simulink model "sim_linear_stateObserver"  (R2020a)
settings: Solver=ode4  StartTime=0.0  StopTime=inf  FixedStep=0.01  RelTol=1e-3
InitFcn:
  | run('initialize_system.m')
values from neighbouring files (symbols this model uses):
  Ac = [d_f1_dth,d_f1_dyw,d_f1_dw_th,d_f1_dw_yw ... (first row only)    [linearize_heli.m]
  Bc = [d_f1_Vmp,d_f1_Vmy ... (first row only)    [linearize_heli.m]
  Cc = [1,0,0,0;0,1,0,0]    [linearize_heli.m]
  th_op = -30*pi/180    (= -0.523598775598)    [initialize_system.m]
  Vmp_op = (Kyy*m_heli*g*cos(th_op)*l_cm) / (Kyy*Kpp - Kyp*Kpy)    [initialize_system.m]
  Vmy_op = (Kyp*Vmp_op) / (Kyy)    [initialize_system.m]
  w_th_op = 0    [initialize_system.m]
  w_yw_op = 0    [initialize_system.m]
  yw_op = pi/2    (= 1.57079632679)    [initialize_system.m]
undefined symbols (not defined in the file or in its folder): L
libraries: realtime_pacer_lib x1
settings Model: Creator=engen  LastModifiedBy=eirik.engen

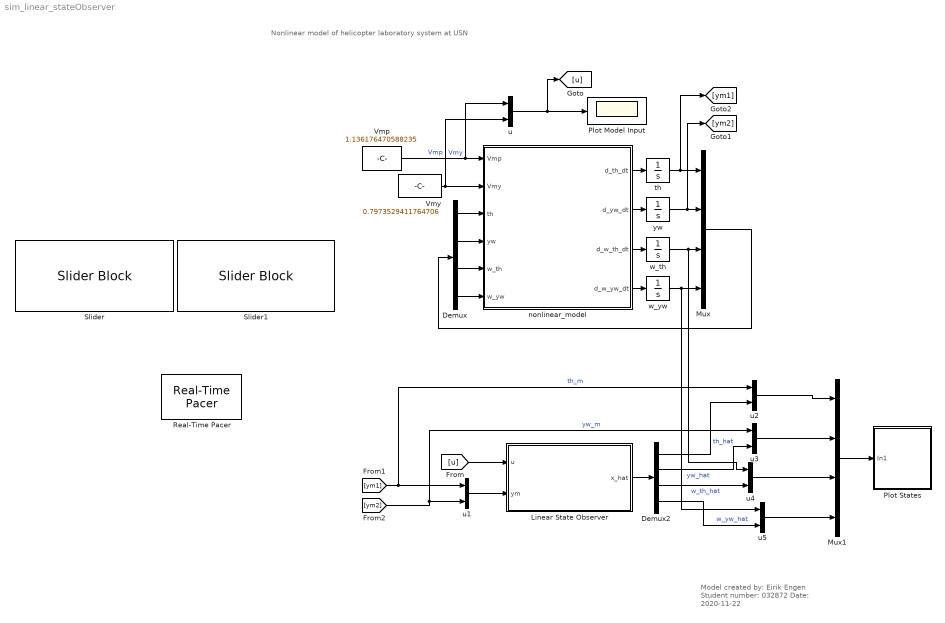
== system sim_linear_stateObserver ==
  note: Model created by: Eirik Engen
      | Student number: 032872
      | Date: 2020-11-22
  note: Nonlinear model of helicopter laboratory system at USN
  Demux : Demux
  Demux2 : Demux
  Linear State Observer : Subsystem
  Mux : Mux
  Mux1 : Mux
  Plot Model Input : Scope
  Plot States : Subsystem
  Real-Time Pacer : realtime_pacer_lib/Real-Time Pacer  simTimePerRealTime=1
      settings: SourceProductName=Real-Time Pacer
  Slider : SliderBlock  ScaleMax=1.6  TickInterval=0.4
  Slider1 : SliderBlock  ScaleMax=1.6  TickInterval=0.4
  Vmp : Constant  Value=1.136176470588235  SampleTime=-1
  Vmy : Constant  Value=0.7973529411764706  SampleTime=-1
  nonlinear_model : MATLAB Function  TreatAsAtomicUnit=on
  th : Integrator  InitialCondition=-10*pi/180  LimitOutput=on  UpperSaturationLimit=45*pi/180  LowerSaturationLimit=-45*pi/180  ContinuousStateAttributes='th'
  u{,1..5} (6 alike) : Mux  Inputs=2
  w_th : Integrator  ContinuousStateAttributes='w_th'
  w_yw : Integrator  ContinuousStateAttributes='w_yw'
  yw : Integrator  InitialCondition=pi/2  LimitOutput=on  UpperSaturationLimit=180*pi/180  LowerSaturationLimit=0  ContinuousStateAttributes='yw'
  wires:
  Vmp/1 -> u/1, nonlinear_model/1(Vmp)  "Vmp"
  Vmy/1 -> u/2, nonlinear_model/2(Vmy)  "Vmy"
  nonlinear_model/1(d_th_dt) -> th/1
  nonlinear_model/2(d_yw_dt) -> yw/1
  nonlinear_model/3(d_w_th_dt) -> w_th/1
  nonlinear_model/4(d_w_yw_dt) -> w_yw/1
  th/1 -> [ym1], Mux/1
  yw/1 -> [ym2], Mux/2
  w_th/1 -> u4/1, Mux/3
  w_yw/1 -> u5/1, Mux/4
  Mux/1 -> Demux/1
  Demux/1 -> nonlinear_model/3(th)
  Demux/2 -> nonlinear_model/4(yw)
  Demux/3 -> nonlinear_model/5(w_th)
  Demux/4 -> nonlinear_model/6(w_yw)
  u/1 -> [u], Plot Model Input/1
  [u] -> Linear State Observer/1(u)
  u1/1 -> Linear State Observer/2(ym)
  Linear State Observer/1(x_hat) -> Demux2/1
  Mux1/1 -> Plot States/1(In1)
  u2/1 -> Mux1/1
  u3/1 -> Mux1/2
  Demux2/1 -> u2/2  "th_hat"
  Demux2/2 -> u3/2  "yw_hat"
  u5/1 -> Mux1/4
  u4/1 -> Mux1/3
  [ym1] -> u2/1, u1/1  "th_m"
  Demux2/4 -> u5/2  "w_yw_hat"
  Demux2/3 -> u4/2  "w_th_hat"
  [ym2] -> u3/1, u1/2  "yw_m"

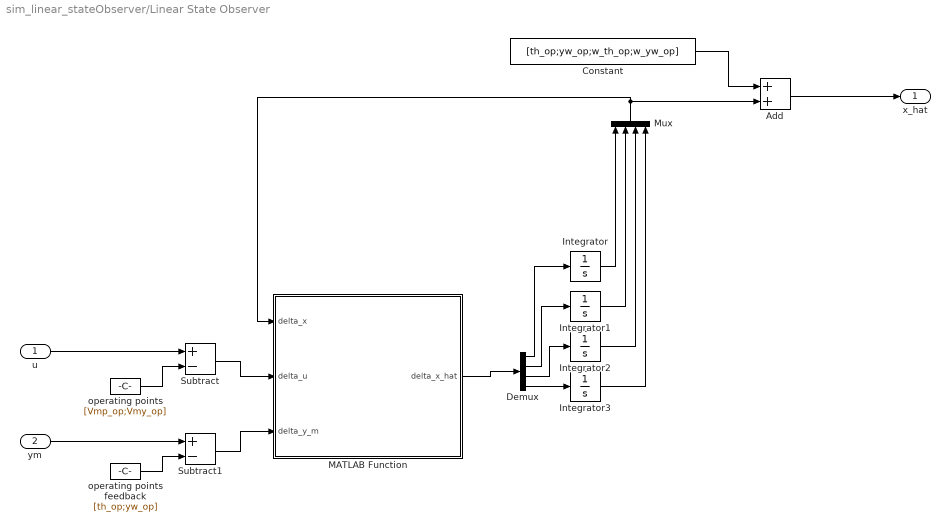
== system sim_linear_stateObserver/Linear State Observer ==
  u : Inport
  ym : Inport  Port=2
  Add : Sum
  Constant : Constant  Value=[th_op;yw_op;w_th_op;w_yw_op]
  Demux : Demux
  Integrator{,1..3} (4 alike) : Integrator
  MATLAB Function : MATLAB Function  TreatAsAtomicUnit=on
  Mux : Mux
  Subtract : Sum  Inputs=+-
  Subtract1 : Sum  Inputs=+-
  operating points : Constant  Value=[Vmp_op;Vmy_op]
  operating points feedback : Constant  Value=[th_op;yw_op]
  x_hat : Outport
  wires:
  MATLAB Function/1(delta_x_hat) -> Demux/1
  u/1 -> Subtract/1
  operating points/1 -> Subtract/2
  Subtract/1 -> MATLAB Function/2(delta_u)
  Mux/1 -> MATLAB Function/1(delta_x), Add/2
  Demux/1 -> Integrator/1
  Demux/2 -> Integrator1/1
  Demux/3 -> Integrator2/1
  Demux/4 -> Integrator3/1
  Integrator/1 -> Mux/1
  Integrator1/1 -> Mux/2
  Integrator2/1 -> Mux/3
  Integrator3/1 -> Mux/4
  Subtract1/1 -> MATLAB Function/3(delta_y_m)
  ym/1 -> Subtract1/1
  operating points feedback/1 -> Subtract1/2
  Constant/1 -> Add/1
  Add/1 -> x_hat/1

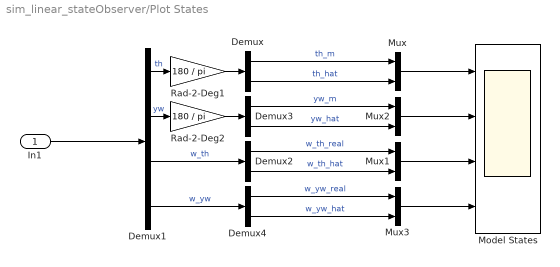
== system sim_linear_stateObserver/Plot States ==
  In1 : Inport
  Demux{,2..4} (4 alike) : Demux  Outputs=2
  Demux1 : Demux
  Model States : Scope  NumInputPorts=4
  Mux{,1..3} (4 alike) : Mux  Inputs=2
  Rad-2-Deg1 : Gain  Gain=180 / pi
  Rad-2-Deg2 : Gain  Gain=180 / pi
  wires:
  In1/1 -> Demux1/1
  Demux/1 -> Mux/1  "th_m"
  Demux/2 -> Mux/2  "th_hat"
  Demux3/1 -> Mux2/1  "yw_m"
  Demux3/2 -> Mux2/2  "yw_hat"
  Demux2/1 -> Mux1/1  "w_th_real"
  Demux2/2 -> Mux1/2  "w_th_hat"
  Demux4/1 -> Mux3/1  "w_yw_real"
  Demux4/2 -> Mux3/2  "w_yw_hat"
  Demux1/1 -> Rad-2-Deg1/1  "th"
  Demux1/2 -> Rad-2-Deg2/1  "yw"
  Demux1/3 -> Demux2/1  "w_th"
  Demux1/4 -> Demux4/1  "w_yw"
  Mux/1 -> Model States/1
  Mux2/1 -> Model States/2
  Mux1/1 -> Model States/3
  Mux3/1 -> Model States/4
  Rad-2-Deg2/1 -> Demux3/1
  Rad-2-Deg1/1 -> Demux/1

== matlab function sim_linear_stateObserver/Linear State Observer/MATLAB Function ==
  data: delta_x input; delta_u input; delta_x_hat output size=4; delta_y_m input; Ac parameter; Bc parameter; Cc parameter; L parameter
function delta_x_hat = linear_state_observer(delta_x, delta_u,delta_y_m,Ac,Bc,Cc,L)
    %apriori state
    delta_x_hat = Ac*delta_x + Bc*delta_u;
    %estimated output    
    y_hat = Cc*delta_x;
    % aposteriori state
    delta_x_hat = delta_x_hat + L*(delta_y_m - y_hat);

== matlab function sim_linear_stateObserver/nonlinear_model ==
  data: Vmp input; d_th_dt output; Vmy input; th input; yw input; w_th input; w_yw input; d_yw_dt output; d_w_th_dt output; d_w_yw_dt output
% Simulink nonlinear model of USN helicopter
% Author: Eirik Engen
% Date: 2020-09-02

function [d_th_dt, d_yw_dt, d_w_th_dt, d_w_yw_dt] = non_linear_model(Vmp, Vmy, th, yw, w_th, w_yw)          %#ok<INUSL>
% function inputs
% Vmp : Model input - Voltage input to Pitch motor/rotor [V]
% Vmy : Model input - Voltage input to Yaw motor/rotor [V]
% th  : Model state - Pitch angle, theta [radians]
% yw  : Model state - Yaw angle, psi [radians]
% w_th: Model state - Pitch angular velocity, omega_theta [radians / s]
% w_yw: Model state - Yaw angular velocity, omega_psi [radians / s]

% System parameters
l_cm   = 0.015;   % [m] - Distance between the pivot point and the center of mass of the helicopter.
m_heli = 0.479;   % [kg] - Total moving mass of the helicopter
J_eq_p = 0.0172;  % [kg-m^2] - Moment of inertia about pitch axis
J_eq_y = 0.0210;  % [kg-m^2] - Moment of inertia about yaw axis
g      = 9.81;    % [m/s^2] - Acceleration due to gravity on planet earth

Kpp    = 0.0556;  % [Nm/V] - Torque constant on pitch axis from pitch motor
Kyy    = 0.21084; % [Nm/V] - Torque constant on yaw axis from yaw motor
Kpy    = 0.005;   % [Nm/V] - Torque constant on pitch axis from yaw motor
Kyp    = 0.15;    % [Nm/V] - Torque constant on yaw axis from pitch motor
Bp     = 0.01;    % [N/V]  - Damping friction factor about pitch axis
By     = 0.08;    % [N/V]  - Damping friction factor about yaw axis

% Differential equations
d_th_dt = w_th;
d_yw_dt = w_yw;
d_w_th_dt = (Kpp*Vmp - ...
    Kpy*Vmy - ...
    Bp*w_th - ...
    m_heli*l_cm^2*w_yw^2*sin(th)*cos(th) - ...
    m_heli*g*l_cm*cos(th)) / ...
    (J_eq_p+m_heli*l_cm^2);
d_w_yw_dt = (Kyp*Vmp - ...
    Kyy*Vmy - ...
    By*w_yw + ...
    2*m_heli*l_cm^2*w_th*w_yw*sin(th)*cos(th)) / ...
    (J_eq_y+m_heli*l_cm^2*cos(th)^2);
